simulink model "sim_closed"  (R2024b)
settings: Solver=VariableStepAuto  StartTime=0.0  StopTime=10.0  RelTol=1e-3
undefined symbols (not defined in the file or in its folder): params
settings Model: Creator=Andre  LastModifiedBy=Andre

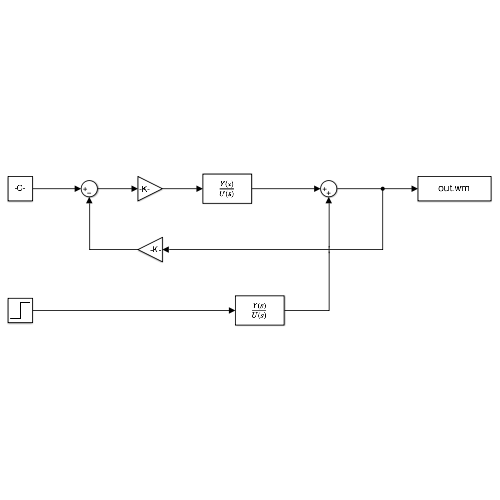
[thumbnail: Simulink's stored preview of the top-level diagram]
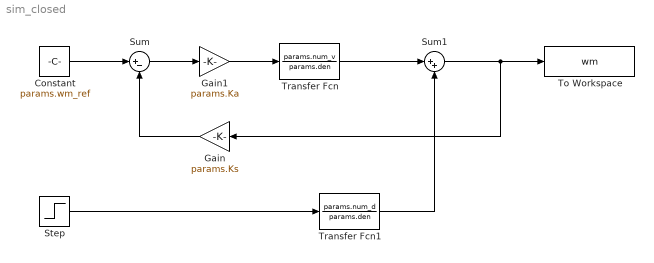
== system sim_closed ==
  Constant : Constant  Value=params.wm_ref
  Gain : Gain  Gain=params.Ks
  Gain1 : Gain  Gain=params.Ka
  Step : Step  Time=params.Td  After=params.TL_step  SampleTime=0
  Sum : Sum  Inputs=|+-
  Sum1 : Sum  Inputs=|++
  To Workspace : ToWorkspace  VariableName=wm  SaveFormat=Timeseries  SampleTime=-1
  Transfer Fcn : TransferFcn  Numerator=params.num_v  Denominator=params.den
  Transfer Fcn1 : TransferFcn  Numerator=params.num_d  Denominator=params.den
  wires:
  Constant/1 -> Sum/1
  Step/1 -> Transfer Fcn1/1
  Sum/1 -> Gain1/1
  Gain1/1 -> Transfer Fcn/1
  Transfer Fcn/1 -> Sum1/1
  Gain/1 -> Sum/2
  Transfer Fcn1/1 -> Sum1/2
  Sum1/1 -> Gain/1, To Workspace/1
